simulink model "ass5_workspace"  (R2020a)
settings: Solver=VariableStepAuto  StartTime=0.0  StopTime=10.0  RelTol=1e-3
values from neighbouring files (symbols this model uses):
  eta = 1    [ass5_run_model.m]
settings Model: Creator=sheld  LastModifiedBy=sheld
settings DebuggingCC: UnderSpecifiedDimensionMsg=warning

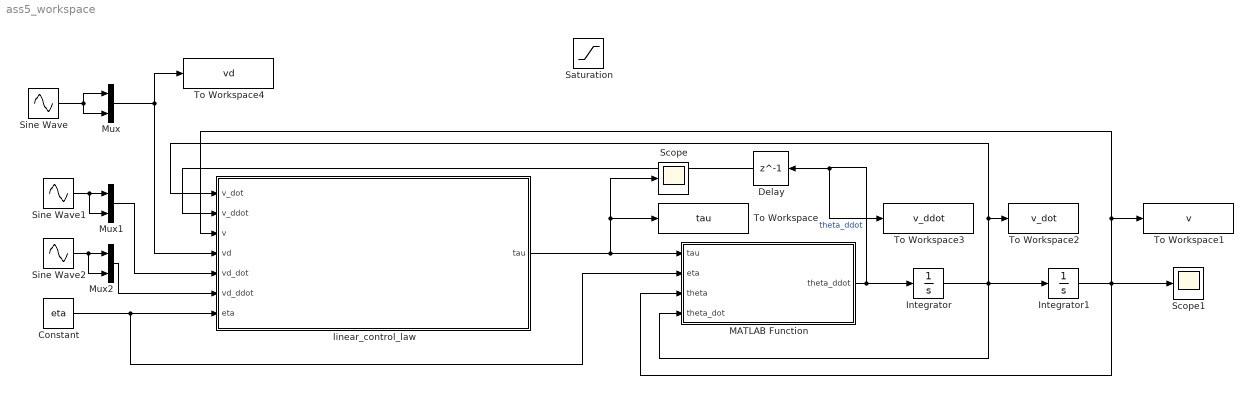
== system ass5_workspace ==
  Constant : Constant  Value=eta
  Delay : Delay  DelayLength=1  InitialCondition=0
  Integrator : Integrator  InitialCondition=[0; 0]
  Integrator1 : Integrator  InitialCondition=[0; 0]
  MATLAB Function : MATLAB Function  TreatAsAtomicUnit=on
  Mux : Mux  Inputs=2
  Mux1 : Mux  Inputs=2
  Mux2 : Mux  Inputs=2
  Saturation : Saturate  UpperLimit=[400; 80]  LowerLimit=[-400; -80]
  Scope : Scope
  Scope1 : Scope
  Sine Wave : Sin  SampleTime=0
  Sine Wave1 : Sin  Phase=pi/2  SampleTime=0
  Sine Wave2 : Sin  Phase=pi  SampleTime=0
  To Workspace : ToWorkspace  VariableName=tau  SampleTime=-1
  To Workspace1 : ToWorkspace  VariableName=v  SampleTime=-1
  To Workspace2 : ToWorkspace  VariableName=v_dot  SampleTime=-1
  To Workspace3 : ToWorkspace  VariableName=v_ddot  SampleTime=-1
  To Workspace4 : ToWorkspace  VariableName=vd  SampleTime=-1
  linear_control_law : MATLAB Function  TreatAsAtomicUnit=on
  wires:
  MATLAB Function/1(theta_ddot) -> To Workspace3/1, Delay/1, Integrator/1  "theta_ddot"
  Integrator/1 -> Integrator1/1, MATLAB Function/4(theta_dot), linear_control_law/1(v_dot), To Workspace2/1
  Constant/1 -> MATLAB Function/2(eta), linear_control_law/7(eta)
  Mux/1 -> To Workspace4/1, linear_control_law/4(vd)
  Sine Wave/1 -> Mux/2, Mux/1
  Sine Wave1/1 -> Mux1/2, Mux1/1
  Mux1/1 -> linear_control_law/5(vd_dot)
  Sine Wave2/1 -> Mux2/2, Mux2/1
  Mux2/1 -> linear_control_law/6(vd_ddot)
  Integrator1/1 -> Scope1/1, To Workspace1/1, linear_control_law/3(v), MATLAB Function/3(theta)
  Delay/1 -> linear_control_law/2(v_ddot)
  linear_control_law/1(tau) -> Scope/1, To Workspace/1, MATLAB Function/1(tau)

== matlab function ass5_workspace/MATLAB Function ==
  data: tau input; eta input; theta input; theta_ddot output; theta_dot input
function theta_ddot = two_link_dyn(tau, eta, theta, theta_dot)

% Static variables

l1 = 0.5;       % L 1
l2 = 0.5;       % L 2
bm1 = 0.1;
bm2 = 0.1;
b1 = 10;          % high
b2 = b1;          % high
a1 = 1;
a2 = 1;
Im1 = 0.2;
Im2 = 0.2;
g = 9.8;
ml1 = 50;         % high  
ml2 = 40;           % high
Iyy1 = b1;        % high
Iyy2 = b1;        % high

I1 = Iyy1 + Iyy2 + ml1*l1*l1 + ml2*(a1^2+l2^2+2*a1*l2*cos(theta(2)));
I2 = Iyy2 + ml2*l2^2;

% Creating the inertia matrix
M11 = I1+eta^2*Im1;
M12 = Iyy2+ml2*(a1*l2*cos(theta(2))+l2^2);
M22 = I2+eta^2*Im2;

%M = [I1+eta^2*Im1 Iyy2+ml2*(a1*l2*c2+l2^2);
%    Iyy2+ml2*(a1*l2*c2+l2^2) I2+eta^2*Im2];

M = 1/eta*[M11 M12;
    M12 M22];

% Creating the inverse of the inertia matrix
det_M = det(M);
M_inv = zeros(2);
M_inv(1,1) = M(2,2);
M_inv(1,2) = -M(2,1);
M_inv(2,1) = M_inv(1,2);
M_inv(2,2) = M(1,1);
M_inv = (1/det_M)*M_inv;

% Creating the gravity vector
G = [(ml1*l1+ml2*l2)*cos(theta(1))*g+(ml2*l2)*cos(theta(1)+theta(2))*g; 
    (ml2*l2)*cos(theta(1)+theta(2))*g];

% Creating the F vector
F = [(b1+eta^2*bm1)*theta_dot(1); 
    (b2+eta^2*bm2)*theta_dot(2)];

% Creating the Coriolis force vector
%V = p(3)*sin(theta(2))*[-theta_dot(2)^2 - 2*theta_dot(1)*theta_dot(2);
%                         theta_dot(1)^2];
V = [-2*ml2*a1*l2*sin(theta(1))*theta_dot(1)*theta_dot(2)-ml2*a1*l2*sin(theta(2))*theta_dot(2)^2;
    ml2*a1*l2*sin(theta(2))*theta_dot(1)^2];
                     
% Calculating the acceleration
theta_ddot = M_inv*(tau + (1/eta)*(- V - F - G));

== matlab function ass5_workspace/linear_control_law ==
  data: v_dot input; v_ddot input; v input; tau output; vd input; vd_dot input; vd_ddot input; eta input
function tau = linear_control(v_dot, v_ddot, v, vd, vd_dot, vd_ddot, eta)

%% Define given constant variables

Iyy1 = 10;
Iyy2 = 10;
Im1 = 0.2;
Im2 = 0.2;
b1 = 10;
b2 = 10;
bm1 = 0.1;
bm2 = 0.1;
ml1 = 50;
ml2 = 40;
l1 = 0.5;
l2 = 0.5;
a1 = 1;
a2 = 1;
g = 9.8;

%% Compute controller parameters

% I1_max = Iyy1 + Iyy2 + ml1*l1^2+ml2*(a1^2+l2^2+2*a1*l2*1);
% I2 = Iyy2 + ml2*l2^2;
% 
% I1_eff_opt = eta*Im1 + (1/eta)*I1_max;
% I2_eff = eta*Im2 + (1/eta)*I2; 
% 
% b1_eff = eta*bm1 + (1/eta)*b1;
% b2_eff = eta*bm2 + (1/eta)*b2;

Kv = 6;
Kp = 9;

%% Compile linear controller

% tau_m_1 = I1_eff_opt*(vd_ddot(1) + Kv*(vd_dot(1)-v_dot(1)) + Kp*(vd(1)-v(1))) + b1_eff*v_dot(1);
% tau_m_2 = I2_eff*(vd_ddot(2) + Kv*(vd_dot(2)-v_dot(2)) + Kp*(vd(2)-v(2))) + b2_eff*v_dot(2);
% tau = [tau_m_1; tau_m_2];

%% Compute nonlinear control

% Gains in matrix form
K_v = [Kv 0; 0 Kv];
K_p = [Kp 0; 0 Kp];

I1 = Iyy1 + Iyy2 + ml1*l1*l1 + ml2*(a1^2+l2^2+2*a1*l2*cos(v(2)));
I2 = Iyy2 + ml2*l2^2;

% M11 = I1+eta^2*Im1;
% M12 = Iyy2+ml2*(a1*l2*cos(v(2))+l2^2);
% M22 = I2+eta^2*Im2;
% M = 1/eta*[M11 M12;
%     M12 M22];
% 
% V = [-2*ml2*a1*l2*sin(v(1))*v_dot(1)*v_dot(2)-ml2*a1*l2*sin(v(2))*v_dot(2)^2;
%     ml2*a1*l2*sin(v(2))*v_dot(1)^2];
% 
% G = [(ml1*l1+ml2*l2)*cos(v(1))*g+(ml2*l2)*cos(v(1)+v(2))*g; 
%     (ml2*l2)*cos(v(1)+v(2))*g];
% 
% F = [(b1+eta^2*bm1)*v_dot(1); 
%     (b2+eta^2*bm2)*v_dot(2)];

M = [82.7+40*cos(v(2)) 20+20*cos(v(2));
    20+20*cos(v(2)) 20.2];

V = [-40*sin(v(2))*v_dot(1)*v_dot(2)-20*sin(v(2))*v_dot(2)^2;
    20*sin(v(2))*v_dot(1)^2];

G = [441*cos(v(1))+196*cos(v(1)+v(2)); 196*cos(v(1)+v(2))];

F = [10.1*v_dot(1); 20*sin(v(2))*v_dot(2)];

% Controller override to try to force high gear to work

% M = [10.0625+cos(v(2)) 0.5+0.5*cos(v(2));
%     0.5+0.5*cos(v(2)) 8.5];
% 
% V = [-sin(v(2))*v_dot(1)*v_dot(2)-0.5*sin(v(2))*v_dot(2)^2;
%     0.5*sin(v(2))*v_dot(1)^2];
% 
% G = [11.025*cos(v(1))+4.9*cos(v(1)+v(2)); 4.9*cos(v(1)+v(2))];
% 
% F = [4.25*v_dot(1); 0.5*sin(v(2))*v_dot(2)];

tau = M*(vd_ddot + K_v*(vd_dot - v_dot) + K_p*(vd - v))+V+G+F;
